simulink subsystem "PieroControladoS"  (R2023b)
settings: Solver=VariableStepAuto  StartTime=0.0  StopTime=10.0  RelTol=1e-3
settings Model: Creator=marqu  LastModifiedBy=marqu

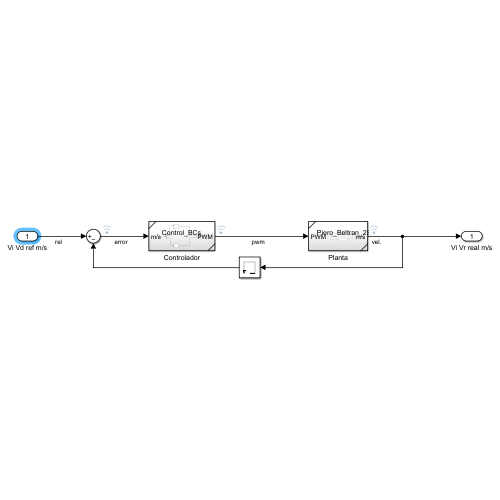
[thumbnail: Simulink's stored preview of the top-level diagram]
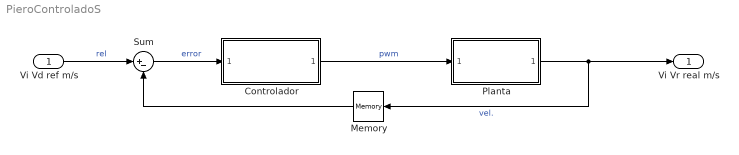
== system PieroControladoS ==
  Vi Vd ref m/s : Inport
  Controlador : Subsystem  ReferencedSubsystem=Control_BCs
  Memory : Memory
  Planta : Subsystem  ReferencedSubsystem=Piero_Beltran_23
  Sum : Sum  Inputs=|+-
  Vi Vr real m/s : Outport
  wires:
  Vi Vd ref m/s/1 -> Sum/1  "rel"
  Sum/1 -> Controlador/1  "error"
  Controlador/1 -> Planta/1  "pwm"
  Planta/1 -> Memory/1, Vi Vr real m/s/1  "vel."
  Memory/1 -> Sum/2
